simulink model "NeuromuscularModel_3R60CMG_3D"  (R2019b)
settings: Solver=ode15s  StartTime=0.0  StopTime=20  MaxStep=.001  MinStep=1e-34  RelTol=1e-5  AbsTol=1e-7  EnableMultiTasking=on
values from neighbouring files (symbols this model uses):
  animFrameRate = 30    [demorun.m]    (also in evaluateCost.m; optimize.m; optimizeCMG.m)
  dt_visual = 1/1000    (= 0.001)    [demorun.m]    (also in evaluateCost.m; optimize.m = 0.0333333333333; optimizeCMG.m)
  initialTargetAngle = 70*pi/180    (= 1.2217304764)    [setInit.m]
  LPreStimBFSHinit = initConditionsSagittal(12)    [assignInit.m]
  LPreStimGASinit = initConditionsSagittal(13)    [assignInit.m]
  LPreStimGLUinit = initConditionsSagittal(8)    [assignInit.m]
  LPreStimHABinit = initConditionsCoronal(6)    [assignInit.m]
  LPreStimHADinit = initConditionsCoronal(7)    [assignInit.m]
  LPreStimHAMinit = initConditionsSagittal(9)    [assignInit.m]
  LPreStimHFLinit = initConditionsSagittal(7)    [assignInit.m]
  LPreStimRFinit = initConditionsSagittal(10)    [assignInit.m]
  LPreStimSOLinit = initConditionsSagittal(14)    [assignInit.m]
  LPreStimTAinit = initConditionsSagittal(15)    [assignInit.m]
  LPreStimVASinit = initConditionsSagittal(11)    [assignInit.m]
  LTargetAngleInit = initConditionsSagittal(6)    [assignInit.m]
  LTargetAngleRInit = initConditionsCoronal(5)    [assignInit.m]
  RPreStimGLUinit = initConditionsSagittal(18)    [assignInit.m]
  RPreStimHABinit = initConditionsCoronal(9)    [assignInit.m]
  RPreStimHADinit = initConditionsCoronal(10)    [assignInit.m]
  RPreStimHAMinit = initConditionsSagittal(19)    [assignInit.m]
  RPreStimHFLinit = initConditionsSagittal(17)    [assignInit.m]
  RPreStimRFinit = initConditionsSagittal(20)    [assignInit.m]
  RTargetAngleInit = initConditionsSagittal(16)    [assignInit.m]
  RTargetAngleRInit = initConditionsCoronal(8)    [assignInit.m]
undefined symbols (not defined in the file or in its folder): DiscIntNeverNeededParam, g, hatLeftHipToCenterDistWidth, LongDelay, LongLoopDelay, MidDelay, ShortDelay, termination_height, thetaHATref, X, Y, Z
libraries: NeuroMuscularLibrary x96, nesl_utility x22, sm_lib x21, CMGlibrary x6, simulink x3
(part 2 of 3)

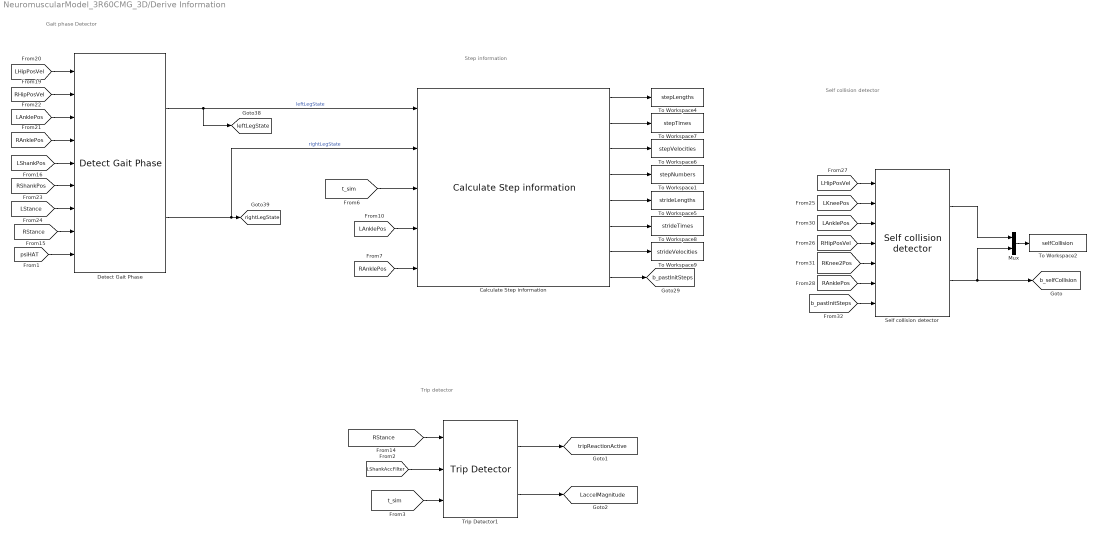
== system NeuromuscularModel_3R60CMG_3D/Derive Information ==
  note: Step information
  note: Self collision detector
  note: Gait phase Detector
  note: Trip detector
  Calculate Step information : NeuroMuscularLibrary/Calculate Step information  SystemSampleTime=-1  Latency=0  AutoFrameSizeCalculation=off
  Detect Gait Phase : NeuroMuscularLibrary/Detect Gait Phase  SystemSampleTime=-1  Latency=0  AutoFrameSizeCalculation=off
  Mux : Mux  Inputs=2
  Self collision detector : NeuroMuscularLibrary/Self collision detector  maxDist=0.02
  To Workspace1 : ToWorkspace  VariableName=stepNumbers  SaveFormat=Structure With Time  SampleTime=-1
  To Workspace2 : ToWorkspace  VariableName=selfCollision  SaveFormat=Structure With Time  SampleTime=dt_visual
  To Workspace4 : ToWorkspace  VariableName=stepLengths  SaveFormat=Structure With Time  SampleTime=-1
  To Workspace5 : ToWorkspace  VariableName=strideLengths  SaveFormat=Structure With Time  SampleTime=-1
  To Workspace6 : ToWorkspace  VariableName=stepVelocities  SaveFormat=Structure With Time  SampleTime=-1
  To Workspace7 : ToWorkspace  VariableName=stepTimes  SaveFormat=Structure With Time  SampleTime=-1
  To Workspace8 : ToWorkspace  VariableName=strideTimes  SaveFormat=Structure With Time  SampleTime=-1
  To Workspace9 : ToWorkspace  VariableName=strideVelocities  SaveFormat=Structure With Time  SampleTime=-1
  Trip Detector1 : CMGlibrary/Trip Detector  tripThreshold=tripDetectThreshold
  tag scope: LaccelMagnitude=global, b_pastInitSteps=global, b_selfCollision=global, leftLegState=global, rightLegState=global, tripReactionActive=global
  wires:
  [RAnklePos] -> Self collision detector/6
  [LAnklePos] -> Self collision detector/3
  Mux/1 -> To Workspace2/1
  [LStance] -> Detect Gait Phase/7
  [LKneePos] -> Self collision detector/2
  [LAnklePos] -> Detect Gait Phase/3
  Self collision detector/1 -> Mux/1
  [RStance] -> Detect Gait Phase/8
  [b_pastInitSteps] -> Self collision detector/7
  [RHipPosVel] -> Self collision detector/4
  Detect Gait Phase/2 -> Calculate Step information/2, [rightLegState]  "rightLegState"
  [LShankPos] -> Detect Gait Phase/5
  [RAnklePos] -> Detect Gait Phase/4
  [RHipPosVel] -> Detect Gait Phase/2
  Detect Gait Phase/1 -> Calculate Step information/1, [leftLegState]  "leftLegState"
  [RShankPos] -> Detect Gait Phase/6
  [LHipPosVel] -> Detect Gait Phase/1
  [psiHAT] -> Detect Gait Phase/9
  [RKnee2Pos] -> Self collision detector/5
  [LHipPosVel] -> Self collision detector/1
  Calculate Step information/1 -> To Workspace4/1
  [RAnklePos] -> Calculate Step information/5
  Calculate Step information/3 -> To Workspace6/1
  Calculate Step information/2 -> To Workspace7/1
  [t_sim] -> Calculate Step information/3
  Calculate Step information/8 -> [b_pastInitSteps]
  [LAnklePos] -> Calculate Step information/4
  Calculate Step information/4 -> To Workspace1/1
  Calculate Step information/5 -> To Workspace5/1
  Calculate Step information/6 -> To Workspace8/1
  Calculate Step information/7 -> To Workspace9/1
  [LShankAccFilter] -> Trip Detector1/2
  [t_sim] -> Trip Detector1/3
  [RStance] -> Trip Detector1/1
  Trip Detector1/1 -> [tripReactionActive]
  Trip Detector1/2 -> [LaccelMagnitude]
  Self collision detector/2 -> [b_selfCollision], Mux/2

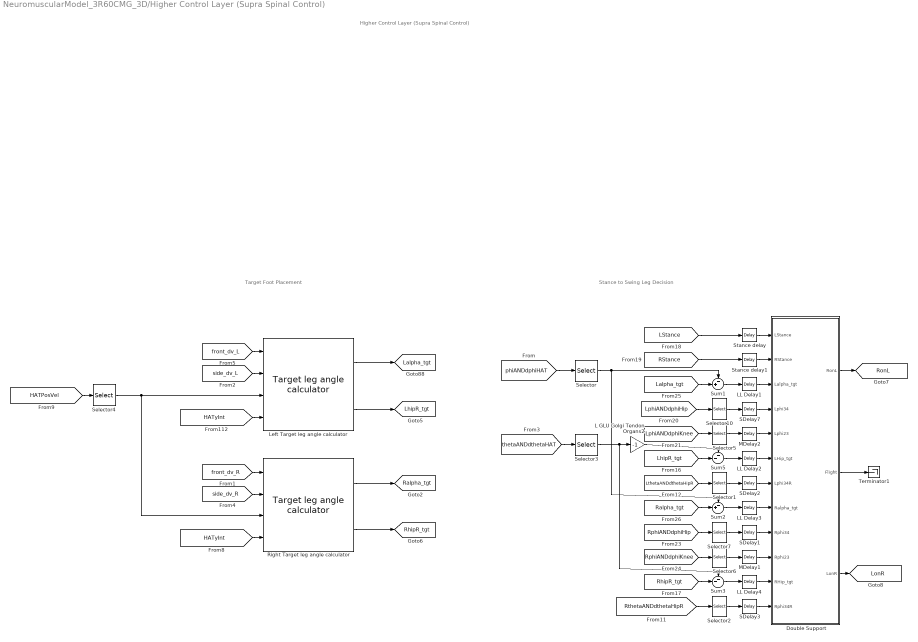
== system NeuromuscularModel_3R60CMG_3D/Higher Control Layer (Supra Spinal Control) ==
  note: Target Foot Placement
  note: Stance to Swing Leg Decision
  note: Higher Control Layer
      | (Supra Spinal Control)
  Double Support : Subsystem
  L GLU Golgi Tendon Organs2 : Gain  Gain=-1
  LL Delay1 : TransportDelay  DelayTime=LongLoopDelay/2  InitialOutput=initialTargetAngle
  LL Delay2 : TransportDelay  DelayTime=LongLoopDelay/2
  LL Delay3 : TransportDelay  DelayTime=LongLoopDelay/2  InitialOutput=initialTargetAngle
  LL Delay4 : TransportDelay  DelayTime=LongLoopDelay/2
  Left Target leg angle calculator : NeuroMuscularLibrary/Target leg angle calculator  simbiconLegAngle0=LsimbiconLegAngle0  simbiconGainD=LsimbiconGainD  simbiconGainV=LsimbiconGainV  simbiconLegAngle0_C=LsimbiconLegAngle0_C  simbiconGainD_C=LsimbiconGainD_C  simbiconGainV_C=LsimbiconGainV_C  headingGain=LheadingGain  headingIntGain=LheadingIntGain
  MDelay1 : TransportDelay  DelayTime=MidDelay
  MDelay2 : TransportDelay  DelayTime=MidDelay
  Right Target leg angle calculator : NeuroMuscularLibrary/Target leg angle calculator  simbiconLegAngle0=RsimbiconLegAngle0  simbiconGainD=RsimbiconGainD  simbiconGainV=RsimbiconGainV  simbiconLegAngle0_C=RsimbiconLegAngle0_C  simbiconGainD_C=RsimbiconGainD_C  simbiconGainV_C=RsimbiconGainV_C  headingGain=RheadingGain  headingIntGain=RheadingIntGain
  SDelay{1..3,7} (4 alike) : TransportDelay  DelayTime=ShortDelay
  Selector : Selector  InputPortWidth=2  IndexOptions=Index vector (dialog)  Indices=[1]  OutputSizes=1
  Selector{1..2,5..7,10} (6 alike) : Selector  InputPortWidth=2  IndexOptions=Index vector (dialog)  Indices=1  OutputSizes=1
  Selector3 : Selector  InputPortWidth=2  IndexOptions=Index vector (dialog)  Indices=[1]  OutputSizes=1
  Selector4 : Selector  InputPortWidth=6  IndexOptions=Index vector (dialog)  Indices=[2]  OutputSizes=1
  Stance delay : TransportDelay  DelayTime=MidDelay
  Stance delay1 : TransportDelay  DelayTime=MidDelay
  Sum1 : Sum  Inputs=-+|
  Sum2 : Sum  Inputs=-+|
  Sum3 : Sum  Inputs=--|
  Sum5 : Sum  Inputs=--|
  Terminator1 : Terminator
  tag scope: Lalpha_tgt=global, LhipR_tgt=global, LonR=global, Ralpha_tgt=global, RhipR_tgt=global, RonL=global
  wires:
  [LphiANDdphiHip] -> Selector10/1
  [LphiANDdphiKnee] -> Selector5/1
  Selector10/1 -> SDelay7/1
  Selector5/1 -> MDelay2/1
  [RphiANDdphiHip] -> Selector7/1
  [RphiANDdphiKnee] -> Selector6/1
  Selector7/1 -> SDelay1/1
  Selector6/1 -> MDelay1/1
  Stance delay/1 -> Double Support/1(LStance)
  Stance delay1/1 -> Double Support/2(RStance)
  [LStance] -> Stance delay/1
  [RStance] -> Stance delay1/1
  Double Support/2(Flight) -> Terminator1/1
  LL Delay1/1 -> Double Support/3(Lalpha_tgt)
  LL Delay3/1 -> Double Support/8(Ralpha_tgt)
  SDelay7/1 -> Double Support/4(Lphi34)
  SDelay1/1 -> Double Support/9(Rphi34)
  MDelay2/1 -> Double Support/5(Lphi23)
  MDelay1/1 -> Double Support/10(Rphi23)
  Sum1/1 -> LL Delay1/1
  [Lalpha_tgt] -> Sum1/2
  Selector/1 -> Sum2/1, Sum1/1
  [Ralpha_tgt] -> Sum2/2
  Sum2/1 -> LL Delay3/1
  [LthetaANDdthetaHipR] -> Selector1/1
  Selector1/1 -> SDelay2/1
  SDelay2/1 -> Double Support/7(Lphi34R)
  LL Delay2/1 -> Double Support/6(LHip_tgt)
  Sum5/1 -> LL Delay2/1
  [LhipR_tgt] -> Sum5/2
  Selector3/1 -> L GLU Golgi Tendon Organs2/1, Sum3/1
  L GLU Golgi Tendon Organs2/1 -> Sum5/1
  [RthetaANDdthetaHipR] -> Selector2/1
  Selector2/1 -> SDelay3/1
  SDelay3/1 -> Double Support/12(Rphi34R)
  LL Delay4/1 -> Double Support/11(RHip_tgt)
  Sum3/1 -> LL Delay4/1
  [RhipR_tgt] -> Sum3/2
  [phiANDdphiHAT] -> Selector/1
  [thetaANDdthetaHAT] -> Selector3/1
  Right Target leg angle calculator/2 -> [RhipR_tgt]
  Right Target leg angle calculator/1 -> [Ralpha_tgt]
  Left Target leg angle calculator/2 -> [LhipR_tgt]
  Left Target leg angle calculator/1 -> [Lalpha_tgt]
  [side_dv_R] -> Right Target leg angle calculator/2
  [side_dv_L] -> Left Target leg angle calculator/2
  [front_dv_R] -> Right Target leg angle calculator/1
  [front_dv_L] -> Left Target leg angle calculator/1
  Double Support/1(RonL) -> [RonL]
  Double Support/3(LonR) -> [LonR]
  [HATyInt] -> Left Target leg angle calculator/4
  [HATyInt] -> Right Target leg angle calculator/4
  [HATPosVel] -> Selector4/1
  Selector4/1 -> Right Target leg angle calculator/3, Left Target leg angle calculator/3

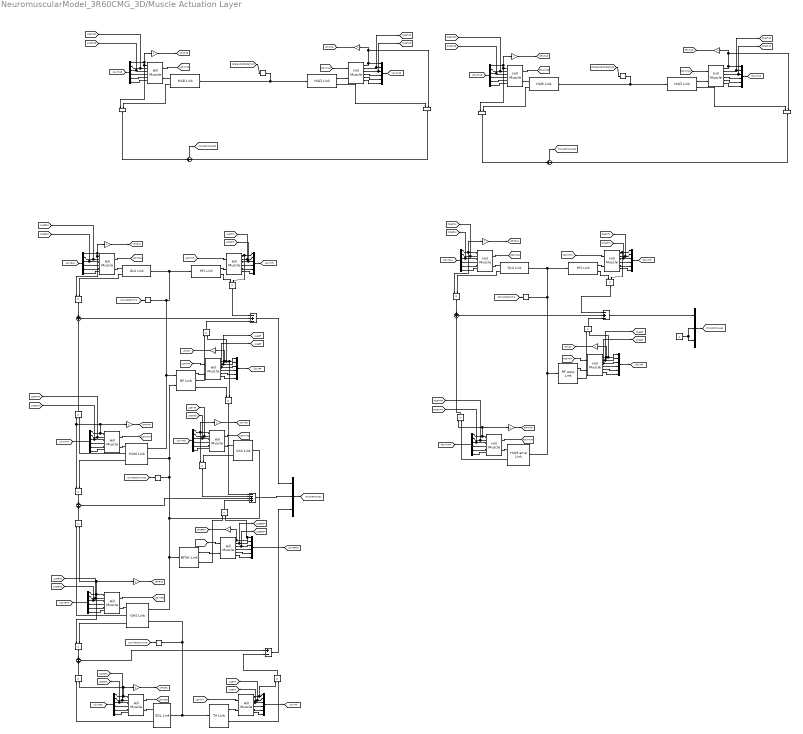
== system NeuromuscularModel_3R60CMG_3D/Muscle Actuation Layer ==
  note: Right Hip Joint
  note: Right Knee Joint
  note: Left Hip Joint
  note: Left Knee Joint
  note: Left Ankle Joint
  note: Left Leg
  note: Right Leg
  note: Body Mechanics Layer
      | Interface (Left Hip Joint)
  note: Muscle Actuation Layer
      | (Coronal Plane)
  note: Muscle Actuation Layer
      | (Sagittal Plane)
  note: Body Mechanics Layer
      | Interface (Right Hip Joint)
  Add1 : Sum  Inputs=-+-
  Add2 : Sum  Inputs=-+-
  Add5 : Sum  Inputs=--++
  Add6 : Sum  Inputs=+-
  Constant : Constant  Value=0
  L  TA Link : NeuroMuscularLibrary/TA Link  SystemSampleTime=-1  Latency=0  AutoFrameSizeCalculation=off
  L BFSH Golgi Tendon Organs : Gain
  L BFSH Link : NeuroMuscularLibrary/BFSH Link  SystemSampleTime=-1  Latency=0  AutoFrameSizeCalculation=off
  L BFSH Muscle : NeuroMuscularLibrary/Hill Muscle  Fmax=FmaxBFSH  lopt=loptBFSH  vmax=vmaxBFSH  lslack=lslackBFSH
  L GAS Golgi Tendon Organs : Gain
  L GAS Link : NeuroMuscularLibrary/GAS Link  SystemSampleTime=-1  Latency=0  AutoFrameSizeCalculation=off
  L GAS Muscle : NeuroMuscularLibrary/Hill Muscle  Fmax=FmaxGAS  lopt=loptGAS  vmax=vmaxGAS  lslack=lslackGAS
  L GLU Golgi Tendon Organs : Gain
  L GLU Link : NeuroMuscularLibrary/GLU Link  SystemSampleTime=-1  Latency=0  AutoFrameSizeCalculation=off
  L GLU Muscle : NeuroMuscularLibrary/Hill Muscle  Fmax=FmaxGLU  lopt=loptGLU  vmax=vmaxGLU  lslack=lslackGLU
  L HAB Golgi Tendon Organs : Gain
  L HAB Link : NeuroMuscularLibrary/HAB Link  SystemSampleTime=-1  Latency=0  AutoFrameSizeCalculation=off
  L HAB Muscle : NeuroMuscularLibrary/Hill Muscle  Fmax=FmaxHAB  lopt=loptHAB  vmax=vmaxHAB  lslack=lslackHAB
  L HAD Golgi Tendon Organs : Gain
  L HAD Link : NeuroMuscularLibrary/HAD Link  SystemSampleTime=-1  Latency=0  AutoFrameSizeCalculation=off
  L HAD Muscle : NeuroMuscularLibrary/Hill Muscle  Fmax=FmaxHAD  lopt=loptHAD  vmax=vmaxHAD  lslack=lslackHAD
  L HAM Golgi Tendon Organs : Gain
  L HAM Link : NeuroMuscularLibrary/HAM Link  SystemSampleTime=-1  Latency=0  AutoFrameSizeCalculation=off
  L HAM Muscle : NeuroMuscularLibrary/Hill Muscle  Fmax=FmaxHAM  lopt=loptHAM  vmax=vmaxHAM  lslack=lslackHAM
  L HFL Link : NeuroMuscularLibrary/HFL Link  SystemSampleTime=-1  Latency=0  AutoFrameSizeCalculation=off
  L HFL Muscle : NeuroMuscularLibrary/Hill Muscle  Fmax=FmaxHFL  lopt=loptHFL  vmax=vmaxHFL  lslack=lslackHFL
  L RF Golgi Tendon Organs : Gain
  L RF Link : NeuroMuscularLibrary/RF Link  SystemSampleTime=-1  Latency=0  AutoFrameSizeCalculation=off
  L RF Muscle : NeuroMuscularLibrary/Hill Muscle  Fmax=FmaxRF  lopt=loptRF  vmax=vmaxRF  lslack=lslackRF
  L SOL Golgi Tendon Organs : Gain
  L SOL Link : NeuroMuscularLibrary/SOL Link  SystemSampleTime=-1  Latency=0  AutoFrameSizeCalculation=off
  L SOL Muscle : NeuroMuscularLibrary/Hill Muscle  Fmax=FmaxSOL  lopt=loptSOL  vmax=vmaxSOL  lslack=lslackSOL
  L TA Muscle : NeuroMuscularLibrary/Hill Muscle  Fmax=FmaxTA  lopt=loptTA  vmax=vmaxTA  lslack=lslackTA
  L VAS Golgi Tendon Organs : Gain
  L VAS Link : NeuroMuscularLibrary/VAS Link  SystemSampleTime=-1  Latency=0  AutoFrameSizeCalculation=off
  L VAS Muscle : NeuroMuscularLibrary/Hill Muscle  Fmax=FmaxVAS  lopt=loptVAS  vmax=vmaxVAS  lslack=lslackVAS
  Mux : Mux  Inputs=3
  Mux1 : Mux  Inputs=3
  Mux{2..10,15..17,19..23} (17 alike) : Mux  Inputs=6
  Product{1..2,26..27} (4 alike) : Product  RndMeth=Zero
  R GLU Golgi Tendon Organs : Gain
  R GLU Link : NeuroMuscularLibrary/GLU Link  SystemSampleTime=-1  Latency=0  AutoFrameSizeCalculation=off
  R GLU amp Muscle : NeuroMuscularLibrary/Hill Muscle  Fmax=FmaxGLUamp  lopt=loptGLUamp  vmax=vmaxGLUamp  lslack=lslackGLUamp
  R HAB Golgi Tendon Organs : Gain
  R HAB Link : NeuroMuscularLibrary/HAB Link  SystemSampleTime=-1  Latency=0  AutoFrameSizeCalculation=off
  R HAB amp Muscle : NeuroMuscularLibrary/Hill Muscle  Fmax=FmaxHABamp  lopt=loptHABamp  vmax=vmaxHABamp  lslack=lslackHABamp
  R HAD Golgi Tendon Organs : Gain
  R HAD Link : NeuroMuscularLibrary/HAD Link  SystemSampleTime=-1  Latency=0  AutoFrameSizeCalculation=off
  R HAD Muscle : NeuroMuscularLibrary/Hill Muscle  Fmax=FmaxHADamp  lopt=loptHADamp  vmax=vmaxHADamp  lslack=lslackHADamp
  R HAM Golgi Tendon Organs : Gain
  R HAM amp Link : NeuroMuscularLibrary/HAM amp Link  SystemSampleTime=-1  Latency=0  AutoFrameSizeCalculation=off
  R HAM amp Muscle : NeuroMuscularLibrary/Hill Muscle  Fmax=FmaxHAMamp  lopt=loptHAMamp  vmax=vmaxHAMamp  lslack=lslackHAMamp
  R HFL  Link : NeuroMuscularLibrary/HFL Link  SystemSampleTime=-1  Latency=0  AutoFrameSizeCalculation=off
  R HFL amp Muscle : NeuroMuscularLibrary/Hill Muscle  Fmax=FmaxHFLamp  lopt=loptHFLamp  vmax=vmaxHFLamp  lslack=lslackHFLamp
  R RF Golgi Tendon Organs : Gain
  R RF amp Link : NeuroMuscularLibrary/RF amp Link  SystemSampleTime=-1  Latency=0  AutoFrameSizeCalculation=off
  R RF amp Muscle : NeuroMuscularLibrary/Hill Muscle  Fmax=FmaxRFamp  lopt=loptRFamp  vmax=vmaxRFamp  lslack=lslackRFamp
  Selector{1,4..8} (6 alike) : Selector  InputPortWidth=2  IndexOptions=Index vector (dialog)  Indices=1  OutputSizes=1
  Sum{1,3..4,8} (4 alike) : Sum  Inputs=+|+
  Sum2 : Sum  Inputs=+-
  Sum25 : Sum  Inputs=+-
  tau = r*F{1..11,18..21,24} (16 alike) : Product
  tag scope: LFmBFSH=global, LFmGAS=global, LFmGLU=global, LFmHAB=global, LFmHAD=global, LFmHAM=global, LFmRF=global, LFmSOL=global, LFmVAS=global, LLceBFSH=global, LLceGAS=global, LLceGLU=global, LLceHAB=global, LLceHAD=global, LLceHAM=global, LLceHFL=global, LLceRF=global, LLceSOL=global, LLceTA=global, LLceVAS=global, LMuscleTorques=global, LMuscleTorquesR=global, LVceBFSH=global, LVceGAS=global, LVceGLU=global, LVceHAB=global, LVceHAD=global, LVceHAM=global, LVceHFL=global, LVceRF=global, LVceSOL=global, LVceTA=global, LVceVAS=global, LdynBFSH=global, LdynGAS=global, LdynGLU=global, LdynHAB=global, LdynHAD=global, LdynHAM=global, LdynHFL=global, LdynRF=global, LdynSOL=global, LdynTA=global, LdynVAS=global, RFmGLU=global, RFmHAB=global, RFmHAD=global, RFmHAM=global, RFmRF=global, RLceGLU=global, RLceHAB=global, RLceHAD=global, RLceHAM=global, RLceHFL=global, RLceRF=global, RMuscleTorques=global, RMuscleTorquesR=global, RVceGLU=global, RVceHAB=global, RVceHAD=global, RVceHAM=global, RVceHFL=global, RVceRF=global, RdynGLU=global, RdynHAB=global, RdynHAD=global, RdynHAM=global, RdynHFL=global, RdynRF=global
  wires:
  R HAM amp Link/1 -> R HAM amp Muscle/2
  R HAM amp Link/2 -> tau = r*F9/2
  R HAM amp Muscle/5 -> Mux7/5
  Mux7/1 -> [RdynHAM]
  R HAM amp Muscle/3 -> [RVceHAM], Mux7/3
  R HAM amp Muscle/4 -> Mux7/4
  [RphiANDdphiHip] -> Selector1/1
  Selector1/1 -> R HAM amp Link/1, R RF amp Link/1, R GLU Link/1, R HFL  Link/1
  Add2/1 -> Mux/1
  R GLU Link/1 -> R GLU amp Muscle/2
  [RStimGLU] -> R GLU amp Muscle/1
  R GLU amp Muscle/5 -> Mux9/5
  R GLU amp Muscle/2 -> [RLceGLU], Mux9/2
  R GLU amp Muscle/3 -> [RVceGLU], Mux9/3
  R GLU amp Muscle/4 -> Mux9/4
  R GLU Link/2 -> tau = r*F10/2
  R GLU amp Muscle/1 -> Mux9/1, R GLU Golgi Tendon Organs/1, tau = r*F10/1
  R GLU Golgi Tendon Organs/1 -> [RFmGLU]
  R HFL  Link/1 -> R HFL amp Muscle/2
  [RStimHFL] -> R HFL amp Muscle/1
  R HFL amp Muscle/5 -> Mux10/5
  Mux10/1 -> [RdynHFL]
  R HFL amp Muscle/4 -> Mux10/4
  R HFL amp Muscle/3 -> [RVceHFL], Mux10/3
  R HFL  Link/2 -> tau = r*F11/1
  R HFL amp Muscle/1 -> Mux10/1, tau = r*F11/2
  R HAM Golgi Tendon Organs/1 -> [RFmHAM]
  [RStimHAM] -> R HAM amp Muscle/1
  tau = r*F9/1 -> Sum8/2  "HAM"
  tau = r*F10/1 -> Sum8/1  "GLU"
  tau = r*F11/1 -> Add2/1  "HFL"
  R HAM amp Muscle/1 -> tau = r*F9/1, R HAM Golgi Tendon Organs/1, Mux7/1
  Sum8/1 -> Add2/2  "Hip Extension Moment"
  Mux9/1 -> [RdynGLU]
  Mux/1 -> [RMuscleTorques]
  L HAM Link/1 -> L HAM Muscle/2
  L HAM Link/2 -> tau = r*F18/2
  L HAM Muscle/5 -> Mux8/5
  Mux8/1 -> [LdynHAM]
  L HAM Muscle/3 -> [LVceHAM], Mux8/3
  L HAM Muscle/4 -> Mux8/4
  [LphiANDdphiHip] -> Selector4/1
  Selector4/1 -> L GLU Link/1, L HFL Link/1, L RF Link/1, L HAM Link/1
  Add1/1 -> Mux1/1
  L GLU Link/1 -> L GLU Muscle/2
  [LStimGLU] -> L GLU Muscle/1
  L GLU Muscle/5 -> Mux15/5
  L GLU Muscle/2 -> Mux15/2, [LLceGLU]
  L GLU Muscle/3 -> Mux15/3, [LVceGLU]
  L GLU Muscle/4 -> Mux15/4
  L GLU Link/2 -> tau = r*F1/2
  L GLU Muscle/1 -> Mux15/1, L GLU Golgi Tendon Organs/1, tau = r*F1/1
  L GLU Golgi Tendon Organs/1 -> [LFmGLU]
  L HFL Link/1 -> L HFL Muscle/2
  [LStimHFL] -> L HFL Muscle/1
  L HFL Muscle/5 -> Mux2/5
  Mux2/1 -> [LdynHFL]
  L HFL Muscle/4 -> Mux2/4
  L HFL Muscle/3 -> [LVceHFL], Mux2/3
  L HFL Link/2 -> tau = r*F2/1
  L HFL Muscle/1 -> Mux2/1, tau = r*F2/2
  L HAM Golgi Tendon Organs/1 -> [LFmHAM]
  [LStimHAM] -> L HAM Muscle/1
  L VAS Link/1 -> L VAS Muscle/2
  L VAS Muscle/5 -> Mux3/5
  Mux3/1 -> [LdynVAS]
  L VAS Muscle/2 -> [LLceVAS], Mux3/2
  L VAS Muscle/3 -> [LVceVAS], Mux3/3
  L VAS Muscle/4 -> Mux3/4
  L VAS Muscle/1 -> L VAS Golgi Tendon Organs/1, Mux3/1, tau = r*F4/1
  L VAS Golgi Tendon Organs/1 -> [LFmVAS]
  L VAS Link/2 -> tau = r*F4/2
  L HAM Link/3 -> tau = r*F5/2
  Sum1/1 -> Add5/3  "Knee Flexion Torque"
  [LStimVAS] -> L VAS Muscle/1
  [LphiANDdphiKnee] -> Selector6/1
  L SOL Muscle/1 -> L SOL Golgi Tendon Organs/1, tau = r*F3/2, Mux5/1
  L SOL Muscle/5 -> Mux5/5
  Mux5/1 -> [LdynSOL]
  L SOL Muscle/3 -> [LVceSOL], Mux5/3
  L SOL Muscle/4 -> Mux5/4
  L SOL Link/2 -> tau = r*F3/1
  L SOL Link/1 -> L SOL Muscle/2
  L SOL Golgi Tendon Organs/1 -> [LFmSOL]
  [LStimSOL] -> L SOL Muscle/1
  Selector5/1 -> L GAS Link/2, L  TA Link/1, L SOL Link/1
  [LphiANDdphiAnkle] -> Selector5/1
  Add6/1 -> Mux1/3
  L  TA Link/1 -> L TA Muscle/2
  L TA Muscle/1 -> tau = r*F6/1, Mux6/1
  L TA Muscle/5 -> Mux6/5
  Mux6/1 -> [LdynTA]
  L TA Muscle/4 -> Mux6/4
  L TA Muscle/3 -> Mux6/3, [LVceTA]
  [LStimTA] -> L TA Muscle/1
  L  TA Link/2 -> tau = r*F6/2
  tau = r*F6/1 -> Add6/2
  L GAS Link/1 -> L GAS Muscle/2
  Selector6/1 -> L GAS Link/1, L BFSH Link/1, L VAS Link/1, L RF Link/2, L HAM Link/2
  L GAS Muscle/5 -> Mux4/5
  Mux4/1 -> [LdynGAS]
  L GAS Muscle/2 -> [LLceGAS], Mux4/2
  L GAS Muscle/3 -> [LVceGAS], Mux4/3
  L GAS Muscle/4 -> Mux4/4
  L GAS Link/2 -> tau = r*F7/1
  [LStimGAS] -> L GAS Muscle/1
  tau = r*F3/1 -> Sum3/2
  Sum3/1 -> Add6/1
  L GAS Link/3 -> tau = r*F8/2
  tau = r*F8/1 -> Sum3/1
  L GAS Muscle/1 -> Mux4/1, tau = r*F7/2, L GAS Golgi Tendon Organs/1, tau = r*F8/1
  L GAS Golgi Tendon Organs/1 -> [LFmGAS]
  tau = r*F18/1 -> Sum4/2  "HAM"
  tau = r*F1/1 -> Sum4/1  "GLU"
  tau = r*F2/1 -> Add1/1  "HFL"
  L HAM Muscle/1 -> tau = r*F5/1, tau = r*F18/1, L HAM Golgi Tendon Organs/1, Mux8/1
  Sum4/1 -> Add1/2  "Hip Extension Moment"
  tau = r*F7/1 -> Sum1/2  "GAS"
  tau = r*F5/1 -> Sum1/1  "HAM"
  tau = r*F4/1 -> Add5/2  "VAS"
  L TA Muscle/2 -> [LLceTA], Mux6/2
  Mux15/1 -> [LdynGLU]
  Mux1/1 -> [LMuscleTorques]
  L GLU Muscle/6 -> Mux15/6
  L HFL Muscle/6 -> Mux2/6
  L HAM Muscle/6 -> Mux8/6
  L VAS Muscle/6 -> Mux3/6
  L GAS Muscle/6 -> Mux4/6
  L SOL Muscle/6 -> Mux5/6
  L TA Muscle/6 -> Mux6/6
  R HAM amp Muscle/6 -> Mux7/6
  R HFL amp Muscle/6 -> Mux10/6
  R GLU amp Muscle/6 -> Mux9/6
  R HFL amp Muscle/2 -> [RLceHFL], Mux10/2
  R HAM amp Muscle/2 -> [RLceHAM], Mux7/2
  L HFL Muscle/2 -> [LLceHFL], Mux2/2
  L HAM Muscle/2 -> [LLceHAM], Mux8/2
  L SOL Muscle/2 -> [LLceSOL], Mux5/2
  L BFSH Muscle/3 -> [LVceBFSH], Mux16/3
  [LStimBFSH] -> L BFSH Muscle/1
  L BFSH Link/2 -> tau = r*F19/1
  L BFSH Golgi Tendon Organs/1 -> [LFmBFSH]
  L BFSH Muscle/6 -> Mux16/6
  L BFSH Muscle/4 -> Mux16/4
  L BFSH Link/1 -> L BFSH Muscle/2
  Mux16/1 -> [LdynBFSH]
  L BFSH Muscle/2 -> [LLceBFSH], Mux16/2
  L BFSH Muscle/5 -> Mux16/5
  L BFSH Muscle/1 -> tau = r*F19/2, Mux16/1, L BFSH Golgi Tendon Organs/1
  tau = r*F19/1 -> Add5/4  "BFSH"
  L RF Muscle/3 -> [LVceRF], Mux17/3
  [LStimRF] -> L RF Muscle/1
  L RF Link/3 -> tau = r*F20/2
  L RF Golgi Tendon Organs/1 -> [LFmRF]
  L RF Muscle/6 -> Mux17/6
  L RF Muscle/4 -> Mux17/4
  L RF Link/1 -> L RF Muscle/2
  Mux17/1 -> [LdynRF]
  L RF Muscle/2 -> [LLceRF], Mux17/2
  L RF Muscle/5 -> Mux17/5
  L RF Muscle/1 -> tau = r*F21/2, Mux17/1, tau = r*F20/1, L RF Golgi Tendon Organs/1
  L RF Link/2 -> tau = r*F21/1
  tau = r*F21/1 -> Add1/3  "RF"
  tau = r*F20/1 -> Add5/1  "RF"
  [RStimRF] -> R RF amp Muscle/1
  R RF amp Muscle/3 -> [RVceRF], Mux19/3
  R RF amp Muscle/4 -> Mux19/4
  R RF amp Muscle/6 -> Mux19/6
  R RF amp Muscle/5 -> Mux19/5
  R RF amp Muscle/2 -> [RLceRF], Mux19/2
  R RF amp Muscle/1 -> tau = r*F24/2, Mux19/1, R RF Golgi Tendon Organs/1
  Mux19/1 -> [RdynRF]
  R RF amp Link/2 -> tau = r*F24/1
  R RF Golgi Tendon Organs/1 -> [RFmRF]
  R RF amp Link/1 -> R RF amp Muscle/2
  tau = r*F24/1 -> Add2/3  "RF"
  Product27/1 -> Sum25/2
  L HAD Link/2 -> Product27/1
  Selector7/1 -> L HAB Link/1, L HAD Link/1
  Product26/1 -> Sum25/1
  L HAB Muscle/6 -> Mux20/6
  L HAB Muscle/1 -> Product26/1, Mux20/1, L HAB Golgi Tendon Organs/1
  L HAB Golgi Tendon Organs/1 -> [LFmHAB]
  L HAB Muscle/4 -> Mux20/4
  L HAB Muscle/2 -> Mux20/2, [LLceHAB]
  L HAB Muscle/5 -> Mux20/5
  L HAB Link/1 -> L HAB Muscle/2
  L HAB Link/2 -> Product26/2
  L HAB Muscle/3 -> Mux20/3, [LVceHAB]
  [LStimHAB] -> L HAB Muscle/1
  Mux20/1 -> [LdynHAB]
  [LthetaANDdthetaHipR] -> Selector7/1
  L HAD Link/1 -> L HAD Muscle/2
  [LStimHAD] -> L HAD Muscle/1
  L HAD Golgi Tendon Organs/1 -> [LFmHAD]
  L HAD Muscle/2 -> Mux21/2, [LLceHAD]
  L HAD Muscle/1 -> Mux21/1, Product27/2, L HAD Golgi Tendon Organs/1
  L HAD Muscle/3 -> [LVceHAD], Mux21/3
  L HAD Muscle/4 -> Mux21/4
  L HAD Muscle/5 -> Mux21/5
  L HAD Muscle/6 -> Mux21/6
  Mux21/1 -> [LdynHAD]
  Sum25/1 -> [LMuscleTorquesR]
  R HAD Muscle/6 -> Mux23/6
  Selector8/1 -> R HAB Link/1, R HAD Link/1
  R HAD Link/2 -> Product2/1
  R HAD Golgi Tendon Organs/1 -> [RFmHAD]
  [RStimHAD] -> R HAD Muscle/1
  Mux23/1 -> [RdynHAD]
  Sum2/1 -> [RMuscleTorquesR]
  Mux22/1 -> [RdynHAB]
  R HAB Golgi Tendon Organs/1 -> [RFmHAB]
  Product1/1 -> Sum2/1
  Product2/1 -> Sum2/2
  R HAD Muscle/5 -> Mux23/5
  R HAD Muscle/2 -> Mux23/2, [RLceHAD]
  R HAD Muscle/3 -> [RVceHAD], Mux23/3
  R HAD Link/1 -> R HAD Muscle/2
  [RthetaANDdthetaHipR] -> Selector8/1
  R HAD Muscle/1 -> Mux23/1, Product2/2, R HAD Golgi Tendon Organs/1
  R HAB Link/2 -> Product1/2
  R HAB amp Muscle/5 -> Mux22/5
  R HAB amp Muscle/2 -> Mux22/2, [RLceHAB]
  R HAD Muscle/4 -> Mux23/4
  R HAB Link/1 -> R HAB amp Muscle/2
  R HAB amp Muscle/4 -> Mux22/4
  R HAB amp Muscle/3 -> Mux22/3, [RVceHAB]
  R HAB amp Muscle/6 -> Mux22/6
  R HAB amp Muscle/1 -> Product1/1, Mux22/1, R HAB Golgi Tendon Organs/1
  [RStimHAB] -> R HAB amp Muscle/1
  Add5/1 -> Mux1/2
  Constant/1 -> Mux/3, Mux/2

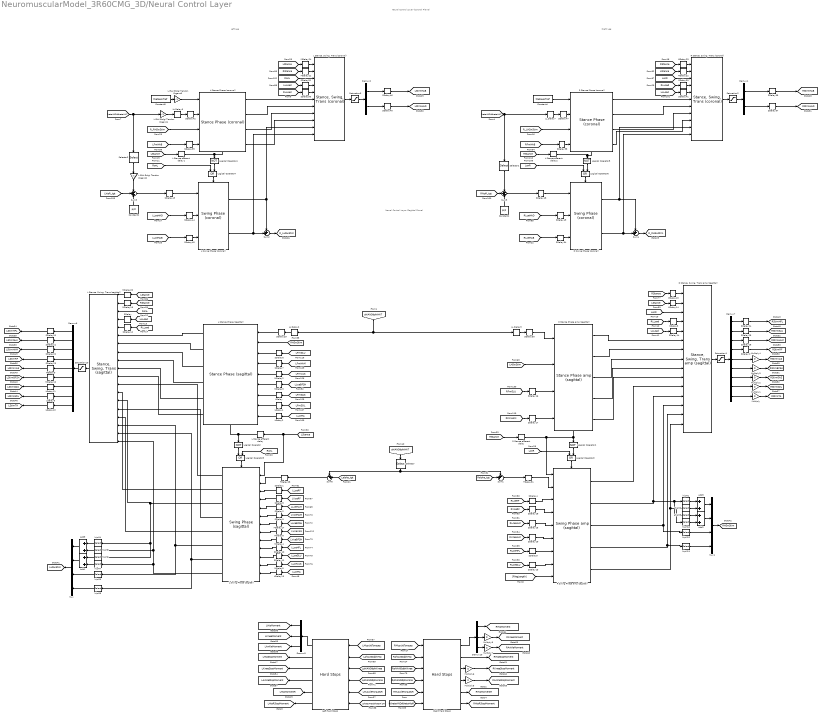
== system NeuromuscularModel_3R60CMG_3D/Neural Control Layer ==
  note: Neural Control Layer
      | (Sagittal Plane)
  note: Neural Control Layer
      | (Coronal Plane)
  note: Right Leg
  note: Left Leg
  Add{1..3,9} (4 alike) : Sum  Inputs=2
  Constant1 : Constant  Value=pi/2
  Constant2 : Constant  Value=pi/2
  Constant3 : Constant  Value=thetaHATref
  Constant4 : Constant  Value=thetaHATref
  Demux1 : Demux  Outputs=2
  Demux10 : Demux  Outputs=3
  Demux2 : Demux  Outputs=2
  Demux6 : Demux  Outputs=9
  Demux7 : Demux  Outputs=9
  Demux8 : Demux  Outputs=3
  L GLU Golgi Tendon Organs1 : Gain  Gain=-1
  L GLU Golgi Tendon Organs2 : Gain  Gain=-1
  L GLU Golgi Tendon Organs3 : Gain  Gain=-1
  L Stance afferent delay : TransportDelay  DelayTime=MidDelay
  L Stance afferent delay1 : TransportDelay  DelayTime=MidDelay
  L Stance afferent delay2 : TransportDelay  DelayTime=MidDelay
  L Stance Phase (coronal) : NeuroMuscularLibrary/Stance Phase (coronal)  PreStimHABst=LPreStimHABst  PreStimHADst=LPreStimHADst  GainFHABst=LGainFHABst  GainPhiHATHABst=LGainPhiHATHABst  GainDphiHATHABst=LGainDphiHATHABst  GainPhiHATHADst=LGainPhiHATHADst  GainDphiHATHADst=LGainDphiHATHADst  GainSHABcHABst=LGainSHABcHABst  GainSHADcHADst=LGainSHADcHADst
  L Stance Phase (sagittal) : NeuroMuscularLibrary/Stance Phase (sagittal)  PreStimHFLst=LPreStimHFLst  PreStimGLUst=LPreStimGLUst  PreStimHAMst=LPreStimHAMst  PreStimRFst=LPreStimRFst  PreStimVASst=LPreStimVASst  PreStimBFSHst=LPreStimBFSHst  PreStimGASst=LPreStimGASst  PreStimSOLst=LPreStimSOLst  PreStimTAst=LPreStimTAst  GainFGLUst=LGainFGLUst  GainFVASst=LGainFVASst  GainFSOLst=LGainFSOLst  GainFHAMst=LGainFHAMst  LceOffsetBFSHVASst=LLceOffsetBFSHVASst  GainLBFSHVASst=LGainLBFSHVASst  LceOffsetBFSHst=LLceOffsetBFSHst  GainLBFSHst=LGainLBFSHst  GainFGASst=LGainFGASst  phiHATref=phiHATref  GainPhiHATHFLst=LGainPhiHATHFLst  GainDphiHATHFLst=LGainDphiHATHFLst  GainPhiHATGLUst=LGainPhiHATGLUst  GainDphiHATGLUst=LGainDphiHATGLUst  GainSGLUHAMst=LGainSGLUHAMst  GainSGLUcHFLst=LGainSGLUcHFLst  GainSHAMcHFLst=LGainSHAMcHFLst  GainSHFLcGLUst=LGainSHFLcGLUst  GainSRFcGLUst=LGainSRFcGLUst  LceOffsetTAst=LLceOffsetTAst  GainLTAst=LGainLTAst  GainFSOLTAst=LGainFSOLTAst
  "L Stance, Swing, Trans (coronal)" : NeuroMuscularLibrary/Stance, Swing, Trans (coronal)  transSupst_C=LtransSupst_C  transsw_C=Ltranssw_C
  "L Stance, Swing, Trans (sagittal)" : NeuroMuscularLibrary/Stance, Swing, Trans (sagittal)  transSupst=LtransSupst  transsw=Ltranssw
  L Swing Phase (coronal) : NeuroMuscularLibrary/Swing Phase (coronal)  PreStimHABsw=LPreStimHABsw  PreStimHADsw=LPreStimHADsw  GainLHABsw=LGainLHABsw  GainLHADsw=LGainLHADsw
  L Swing Phase (sagittal) : NeuroMuscularLibrary/Swing Phase (sagittal)  PreStimHFLsw=LPreStimHFLsw  PreStimGLUsw=LPreStimGLUsw  PreStimHAMsw=LPreStimHAMsw  PreStimRFsw=LPreStimRFsw  PreStimVASsw=LPreStimVASsw  PreStimBFSHsw=LPreStimBFSHsw  PreStimGASsw=LPreStimGASsw  PreStimSOLsw=LPreStimSOLsw  PreStimTAsw=LPreStimTAsw  GainLTAsw=LGainLTAsw  LceOffsetTAsw=LLceOffsetTAsw  GainLRFHFLsw=LGainLRFHFLsw  GainVRFHFLsw=LGainVRFHFLsw  GainLHAMGLUsw=LGainLHAMGLUsw  GainVHAMGLUsw=LGainVHAMGLUsw  GainVRFBFSHsw=LGainVRFBFSHsw  GainVVASRFsw=LGainVVASRFsw  GainVBFSHsw=LGainVBFSHsw  GainLHAMsw=LGainLHAMsw  GainSHAMBFSHsw=LGainSHAMBFSHsw  GainSHAMGASsw=LGainSHAMGASsw  SHAMthresholdsw=LSHAMthresholdsw  GainLHFLsw=LGainLHFLsw  GainLGLUsw=LGainLGLUsw  LceOffsetVASsw=LLceOffsetVASsw  GainLVASsw=LGainLVASsw  legLengthClr=LlegLengthClr  deltaLegAngleThr=LdeltaLegAngleThr
  LDelay : TransportDelay  DelayTime=LongDelay
  LDelay1 : TransportDelay  DelayTime=LongDelay
  LDelay10 : TransportDelay  DelayTime=LongDelay  InitialOutput=LPreStimTAinit
  LDelay11 : TransportDelay  DelayTime=LongDelay  InitialOutput=LPreStimGASinit
  LDelay13 : TransportDelay  DelayTime=LongDelay  InitialOutput=1
  LDelay2 : TransportDelay  DelayTime=LongDelay  InitialOutput=1
  LDelay9 : TransportDelay  DelayTime=LongDelay  InitialOutput=LPreStimSOLinit
  LL Delay{2..3,6..7} (4 alike) : TransportDelay  DelayTime=LongLoopDelay/2
  Left Hard Stops : NeuroMuscularLibrary/Hard Stops  SystemSampleTime=-1  Latency=0  AutoFrameSizeCalculation=off
  Logical Operator{,1,4..5} (4 alike) : Logic  Operator=NOT  AllPortsSameDT=off  OutDataTypeStr=boolean
  Logical Operator{2..3,6..7} (4 alike) : Logic  Operator=OR  AllPortsSameDT=off  OutDataTypeStr=boolean
  MDelay10 : TransportDelay  DelayTime=MidDelay  InitialOutput=LPreStimBFSHinit
  MDelay{2,4,8,13..14,19..24} (11 alike) : TransportDelay  DelayTime=MidDelay
  MDelay17 : TransportDelay  DelayTime=MidDelay  InitialOutput=1
  MDelay3 : TransportDelay  DelayTime=MidDelay  InitialOutput=1
  MDelay5 : TransportDelay  DelayTime=MidDelay  InitialOutput=1
  MDelay9 : TransportDelay  DelayTime=MidDelay  InitialOutput=LPreStimVASinit
  Multiply{,1..8} (9 alike) : Gain  Gain=0
  Mux : Mux
  Mux1 : Mux
  R Stance afferent delay : TransportDelay  DelayTime=MidDelay
  R Stance Phase (coronal) : NeuroMuscularLibrary/Stance Phase (coronal)  PreStimHABst=RPreStimHABst  PreStimHADst=RPreStimHADst  GainFHABst=RGainFHABst  GainPhiHATHABst=RGainPhiHATHABst  GainDphiHATHABst=RGainDphiHATHABst  GainPhiHATHADst=RGainPhiHATHADst  GainDphiHATHADst=RGainDphiHATHADst  GainSHABcHABst=RGainSHABcHABst  GainSHADcHADst=RGainSHADcHADst
  R Stance Phase amp (sagittal) : NeuroMuscularLibrary/Stance Phase amp (sagittal)  PreStimHFLst=RPreStimHFLst  PreStimGLUst=RPreStimGLUst  PreStimHAMst=RPreStimHAMst  PreStimRFst=RPreStimRFst  GainFGLUst=RGainFGLUst  GainFHAMst=RGainFHAMst  phiHATref=phiHATref  GainPhiHATHFLst=RGainPhiHATHFLst  GainDphiHATHFLst=RGainDphiHATHFLst  GainPhiHATGLUst=RGainPhiHATGLUst  GainDphiHATGLUst=RGainDphiHATGLUst  GainSGLUHAMst=RGainSGLUHAMst  GainSGLUcHFLst=RGainSGLUcHFLst  GainSHAMcHFLst=RGainSHAMcHFLst  GainSHFLcGLUst=RGainSHFLcGLUst  GainSRFcGLUst=RGainSRFcGLUst
  "R Stance, Swing, Trans (coronal)" : NeuroMuscularLibrary/Stance, Swing, Trans (coronal)  transSupst_C=RtransSupst_C  transsw_C=Rtranssw_C
  "R Stance, Swing, Trans amp (sagittal)" : NeuroMuscularLibrary/Stance, Swing, Trans amp (sagittal)  transSupst=RtransSupst  transsw=Rtranssw
  R Swing Phase (coronal) : NeuroMuscularLibrary/Swing Phase (coronal)  PreStimHABsw=RPreStimHABsw  PreStimHADsw=RPreStimHADsw  GainLHABsw=RGainLHABsw  GainLHADsw=RGainLHADsw
  R Swing Phase amp (sagittal) : NeuroMuscularLibrary/Swing Phase amp (sagittal)  PreStimHFLsw=RPreStimHFLsw  PreStimGLUsw=RPreStimGLUsw  PreStimHAMsw=RPreStimHAMsw  PreStimRFsw=RPreStimRFsw  GainLRFHFLsw=RGainLRFHFLsw  GainVRFHFLsw=RGainVRFHFLsw  GainLHAMGLUsw=RGainLHAMGLUsw  GainVHAMGLUsw=RGainVHAMGLUsw  GainLHAMsw=RGainLHAMsw  GainLHFLsw=RGainLHFLsw  GainLGLUsw=RGainLGLUsw  legLengthClr=RlegLengthClr  deltaLegAngleThr=RdeltaLegAngleThr
  Right Hard Stops : NeuroMuscularLibrary/Hard Stops  SystemSampleTime=-1  Latency=0  AutoFrameSizeCalculation=off
  SDelay{,3,6..9,12,14,16..19,29..30,32..33,36,38..39,41..42,47} (22 alike) : TransportDelay  DelayTime=ShortDelay
  SDelay{1..2,4..5,10..11,13,15,34,44..45,49} (12 alike) : TransportDelay  DelayTime=ShortDelay  InitialOutput=1
  SDelay20 : TransportDelay  DelayTime=ShortDelay  InitialOutput=LPreStimHFLinit
  SDelay21 : TransportDelay  DelayTime=ShortDelay  InitialOutput=LPreStimGLUinit
  SDelay22 : TransportDelay  DelayTime=ShortDelay  InitialOutput=LPreStimHAMinit
  SDelay23 : TransportDelay  DelayTime=ShortDelay  InitialOutput=LPreStimRFinit
  SDelay24 : TransportDelay  DelayTime=ShortDelay  InitialOutput=RPreStimHFLinit
  SDelay25 : TransportDelay  DelayTime=ShortDelay  InitialOutput=RPreStimGLUinit
  SDelay26 : TransportDelay  DelayTime=ShortDelay  InitialOutput=RPreStimHAMinit
  SDelay27 : TransportDelay  DelayTime=ShortDelay  InitialOutput=RPreStimRFinit
  SDelay35 : TransportDelay  DelayTime=ShortDelay  InitialOutput=RPreStimHABinit
  SDelay37 : TransportDelay  DelayTime=ShortDelay  InitialOutput=RPreStimHADinit
  SDelay40 : TransportDelay  DelayTime=ShortDelay  InitialOutput=LPreStimHADinit
  SDelay43 : TransportDelay  DelayTime=(ShortDelay + LongLoopDelay/2)  InitialOutput=LTargetAngleRInit
  SDelay46 : TransportDelay  DelayTime=ShortDelay  InitialOutput=LPreStimHABinit
  SDelay48 : TransportDelay  DelayTime=(ShortDelay + LongLoopDelay/2)  InitialOutput=RTargetAngleRInit
  Saturation{1..3,10} (4 alike) : Saturate  UpperLimit=1  LowerLimit=0.01  ZeroCross=off
  Selector : Selector  InputPortWidth=2  IndexOptions=Index vector (dialog)  Indices=[1]  OutputSizes=1
  Selector1 : Selector  InputPortWidth=2  IndexOptions=Index vector (dialog)  Indices=[1]  OutputSizes=1
  Selector2 : Selector  InputPortWidth=2  IndexOptions=Index vector (dialog)  Indices=[1]  OutputSizes=1
  Sum1 : Sum  Inputs=-+|
  Sum2 : Sum  Inputs=++|
  Sum3 : Sum  Inputs=--+
  Sum4 : Sum  Inputs=++|
  Sum5 : Sum  Inputs=--+
  Sum6 : Sum  Inputs=-+|
  TDelay28 : TransportDelay  DelayTime=(ShortDelay + LongLoopDelay/2)  InitialOutput=LTargetAngleInit
  TDelay31 : TransportDelay  DelayTime=(ShortDelay + LongLoopDelay/2)  InitialOutput=RTargetAngleInit
  hipM{1,4,9,12} (4 alike) : Selector  InputPortWidth=2  IndexOptions=Index vector (dialog)  Indices=1  OutputSizes=1
  hipM10 : Selector  InputPortWidth=3  IndexOptions=Index vector (dialog)  Indices=2  OutputSizes=1
  hipM{2,5,8,11} (4 alike) : Selector  InputPortWidth=3  IndexOptions=Index vector (dialog)  Indices=1  OutputSizes=1
  hipM3 : Selector  InputPortWidth=2  IndexOptions=Index vector (dialog)  Indices=2  OutputSizes=1
  hipM6 : Selector  InputPortWidth=2  IndexOptions=Index vector (dialog)  Indices=2  OutputSizes=1
  hipM7 : Selector  InputPortWidth=3  IndexOptions=Index vector (dialog)  Indices=2  OutputSizes=1
  tag scope: LAnkleMoment=global, LAnkleStopMoment=global, LHSwStim=global, LHipMoment=global, LHipMomentR=global, LHipRStopMoment=global, LHipStopMoment=global, LKneeMoment=global, LKneeStopMoment=global, LStimBFSH=global, LStimGAS=global, LStimGLU=global, LStimHAB=global, LStimHAD=global, LStimHAM=global, LStimHFL=global, LStimRF=global, LStimSOL=global, LStimTA=global, LStimVAS=global, RAnkleMoment=global, RAnkleStopMoment=global, RHSwStim=global, RHipMoment=global, RHipMomentR=global, RHipRStopMoment=global, RHipStopMoment=global, RKneeMoment=global, RKneeStopMoment=global, RStimBFSH=global, RStimGAS=global, RStimGLU=global, RStimHAB=global, RStimHAD=global, RStimHAM=global, RStimHFL=global, RStimRF=global, RStimSOL=global, RStimTA=global, RStimVAS=global, R_LHSwStim=global, R_RHSwStim=global
  wires:
  L Swing Phase (sagittal)/7 -> "L Stance, Swing, Trans (sagittal)"/18, hipM8/1
  Mux/1 -> [LHSwStim]
  hipM2/1 -> Add3/2
  SDelay11/1 -> L Swing Phase (sagittal)/11
  [RLceRF] -> SDelay4/1
  MDelay19/1 -> "L Stance, Swing, Trans (sagittal)"/2
  SDelay10/1 -> L Swing Phase (sagittal)/10
  hipM10/1 -> Add2/2
  R Stance Phase amp (sagittal)/5 -> "R Stance, Swing, Trans amp (sagittal)"/10
  hipM4/1 -> Add9/1
  SDelay2/1 -> L Swing Phase (sagittal)/5
  [RLceGLU] -> SDelay13/1
  L Swing Phase (sagittal)/1 -> "L Stance, Swing, Trans (sagittal)"/12
  LDelay/1 -> L Stance Phase (sagittal)/7
  L Stance Phase (sagittal)/1 -> "L Stance, Swing, Trans (sagittal)"/6
  SDelay9/1 -> L Swing Phase (sagittal)/6
  L Swing Phase (sagittal)/3 -> "L Stance, Swing, Trans (sagittal)"/14, hipM6/1, hipM4/1
  R Swing Phase amp (sagittal)/4 -> "R Stance, Swing, Trans amp (sagittal)"/14, hipM11/1
  Add2/1 -> Mux1/2
  L Swing Phase (sagittal)/5 -> "L Stance, Swing, Trans (sagittal)"/16
  SDelay14/1 -> "R Stance, Swing, Trans amp (sagittal)"/5
  R Stance Phase amp (sagittal)/2 -> "R Stance, Swing, Trans amp (sagittal)"/7
  SDelay12/1 -> "L Stance, Swing, Trans (sagittal)"/5
  MDelay2/1 -> L Stance Phase (sagittal)/5
  hipM6/1 -> Add1/1
  R Stance Phase amp (sagittal)/3 -> "R Stance, Swing, Trans amp (sagittal)"/8
  L Stance Phase (sagittal)/6 -> "L Stance, Swing, Trans (sagittal)"/11
  SDelay4/1 -> R Swing Phase amp (sagittal)/3
  hipM11/1 -> Mux1/4
  MDelay8/1 -> L Swing Phase (sagittal)/8
  Add3/1 -> Mux1/1
  R Swing Phase amp (sagittal)/3 -> "R Stance, Swing, Trans amp (sagittal)"/13, hipM12/1
  "R Stance, Swing, Trans amp (sagittal)"/1 -> Saturation1/1
  Add1/1 -> Mux/2
  hipM9/1 -> Mux/3
  L Stance Phase (sagittal)/3 -> "L Stance, Swing, Trans (sagittal)"/8
  Demux7/8 -> Multiply1/1
  Logical Operator2/1 -> R Swing Phase amp (sagittal)/Enable
  hipM5/1 -> Add9/2
  MDelay20/1 -> "L Stance, Swing, Trans (sagittal)"/1
  L Swing Phase (sagittal)/2 -> "L Stance, Swing, Trans (sagittal)"/13
  hipM8/1 -> Mux/4
  L Swing Phase (sagittal)/4 -> "L Stance, Swing, Trans (sagittal)"/15
  L Swing Phase (sagittal)/8 -> "L Stance, Swing, Trans (sagittal)"/19, hipM5/1, hipM7/1
  [LStance] -> MDelay20/1
  R Stance Phase amp (sagittal)/4 -> "R Stance, Swing, Trans amp (sagittal)"/9
  LL Delay3/1 -> SDelay30/1
  SDelay30/1 -> R Stance Phase amp (sagittal)/1
  SDelay29/1 -> L Stance Phase (sagittal)/1
  hipM1/1 -> Add3/1
  R Swing Phase amp (sagittal)/5 -> "R Stance, Swing, Trans amp (sagittal)"/15, hipM2/1, hipM10/1
  [LLceGLU] -> SDelay11/1
  [RLceHFL] -> SDelay5/1
  L Stance Phase (sagittal)/2 -> "L Stance, Swing, Trans (sagittal)"/7
  R Stance Phase amp (sagittal)/1 -> "R Stance, Swing, Trans amp (sagittal)"/6
  [LLceVAS] -> MDelay5/1
  [LHSwStim] -> R Stance Phase amp (sagittal)/2
  SDelay/1 -> "L Stance, Swing, Trans (sagittal)"/4
  Demux7/6 -> Multiply3/1
  Add9/1 -> Mux/1
  [LLceHFL] -> SDelay10/1
  [LLLoad] -> SDelay14/1
  Saturation1/1 -> Demux7/1
  SDelay5/1 -> R Swing Phase amp (sagittal)/7
  [LFmSOL] -> LDelay1/1
  hipM12/1 -> Mux1/3
  [LonR] -> "R Stance, Swing, Trans amp (sagittal)"/3
  [LLLoad] -> SDelay/1
  L Stance Phase (sagittal)/4 -> "L Stance, Swing, Trans (sagittal)"/9
  hipM3/1 -> Add2/1
  R Swing Phase amp (sagittal)/1 -> "R Stance, Swing, Trans amp (sagittal)"/11
  L Stance Phase (sagittal)/5 -> "L Stance, Swing, Trans (sagittal)"/10
  SDelay3/1 -> "R Stance, Swing, Trans amp (sagittal)"/4
  SDelay19/1 -> R Swing Phase amp (sagittal)/6
  [RVceHAM] -> SDelay19/1
  SDelay18/1 -> R Swing Phase amp (sagittal)/4
  SDelay15/1 -> R Swing Phase amp (sagittal)/5
  [RLceHAM] -> SDelay15/1
  Demux7/7 -> Multiply2/1
  [LLceBFSH] -> MDelay3/1
  [RLLoad] -> SDelay3/1
  SDelay17/1 -> R Stance Phase amp (sagittal)/4
  [RStance] -> MDelay19/1
  MDelay4/1 -> L Swing Phase (sagittal)/9
  L Swing Phase (sagittal)/6 -> "L Stance, Swing, Trans (sagittal)"/17, hipM9/1
  Demux7/9 -> Multiply/1
  [LVceBFSH] -> MDelay4/1
  SDelay8/1 -> L Swing Phase (sagittal)/4
  [RVceRF] -> SDelay18/1
  MDelay5/1 -> L Swing Phase (sagittal)/12
  SDelay16/1 -> R Stance Phase amp (sagittal)/3
  [RLLoad] -> SDelay12/1
  R Swing Phase amp (sagittal)/2 -> "R Stance, Swing, Trans amp (sagittal)"/12, hipM3/1, hipM1/1
  [LVceRF] -> SDelay8/1
  SDelay13/1 -> R Swing Phase amp (sagittal)/8
  Mux1/1 -> [RHSwStim]
  L Stance afferent delay/1 -> L Stance Phase (sagittal)/Enable, Logical Operator/1
  Logical Operator3/1 -> L Swing Phase (sagittal)/Enable
  [LLceRF] -> SDelay1/1
  [LVceHAM] -> SDelay9/1
  LDelay2/1 -> L Stance Phase (sagittal)/9
  [LLceTA] -> LDelay2/1
  SDelay1/1 -> L Swing Phase (sagittal)/3
  [RFmHAM] -> SDelay17/1
  Logical Operator/1 -> Logical Operator3/2
  [LLceHAM] -> SDelay2/1
  LDelay1/1 -> L Stance Phase (sagittal)/8
  [LFmGAS] -> LDelay/1
  [RFmGLU] -> SDelay16/1
  MDelay3/1 -> L Stance Phase (sagittal)/6
  SDelay6/1 -> L Stance Phase (sagittal)/3
  [LVceVAS] -> MDelay8/1
  [LFmVAS] -> MDelay2/1
  LL Delay2/1 -> SDelay29/1
  [LFmGLU] -> SDelay6/1
  SDelay7/1 -> L Stance Phase (sagittal)/4
  Demux7/5 -> Multiply4/1
  [LFmHAM] -> SDelay7/1
  [RHSwStim] -> L Stance Phase (sagittal)/2
  hipM7/1 -> Add1/2
  Logical Operator1/1 -> Logical Operator2/2
  [LLceTA] -> LDelay13/1
  MDelay17/1 -> L Swing Phase (sagittal)/7
  [LLceBFSH] -> MDelay17/1
  LDelay13/1 -> L Swing Phase (sagittal)/13
  R Stance afferent delay/1 -> R Swing Phase amp (sagittal)/1, R Stance Phase amp (sagittal)/Enable, Logical Operator1/1
  [RonL] -> "L Stance, Swing, Trans (sagittal)"/3
  [LonR] -> Logical Operator2/1
  [RonL] -> Logical Operator3/1
  [RStance] -> MDelay13/1
  MDelay13/1 -> "R Stance, Swing, Trans amp (sagittal)"/1
  [LStance] -> MDelay14/1
  MDelay14/1 -> "R Stance, Swing, Trans amp (sagittal)"/2
  [Ralpha_tgt] -> Sum1/2
  Selector/1 -> Sum6/1, Sum1/1
  [Lalpha_tgt] -> Sum6/2
  [phiANDdphiHAT] -> LL Delay2/1, LL Delay3/1
  [RFmHAB] -> SDelay38/1
  SDelay35/1 -> [RStimHAB]
  [LFmHAB] -> SDelay39/1
  SDelay37/1 -> [RStimHAD]
  [LLceHAD] -> SDelay44/1
  SDelay39/1 -> L Stance Phase (coronal)/4
  L Stance Phase (coronal)/2 -> "L Stance, Swing, Trans (coronal)"/7
  MDelay21/1 -> "L Stance, Swing, Trans (coronal)"/2
  L Swing Phase (coronal)/2 -> "L Stance, Swing, Trans (coronal)"/11, Sum2/2
  [LhipR_tgt] -> Sum3/2
  L GLU Golgi Tendon Organs2/1 -> Sum3/1
  Logical Operator5/1 -> Logical Operator6/2
  [RLceHAD] -> SDelay49/1
  Selector2/1 -> L GLU Golgi Tendon Organs2/1
  Logical Operator4/1 -> Logical Operator7/2
  [LLceHAB] -> SDelay45/1
  Constant4/1 -> R Stance Phase (coronal)/1
  [RonL] -> Logical Operator7/1
  Logical Operator6/1 -> R Swing Phase (coronal)/Enable
  L Swing Phase (coronal)/1 -> "L Stance, Swing, Trans (coronal)"/10, Sum2/1
  L Stance Phase (coronal)/1 -> "L Stance, Swing, Trans (coronal)"/6
  SDelay32/1 -> "L Stance, Swing, Trans (coronal)"/4
  L GLU Golgi Tendon Organs1/1 -> LL Delay6/1
  "L Stance, Swing, Trans (coronal)"/1 -> Saturation3/1
  SDelay43/1 -> L Swing Phase (coronal)/1
  MDelay24/1 -> "L Stance, Swing, Trans (coronal)"/1
  Selector1/1 -> Sum5/1
  L Stance afferent delay1/1 -> Logical Operator4/1, L Stance Phase (coronal)/Enable
  SDelay46/1 -> [LStimHAB]
  Sum3/1 -> SDelay43/1
  SDelay45/1 -> L Swing Phase (coronal)/3
  SDelay44/1 -> L Swing Phase (coronal)/2
  [RStance] -> MDelay23/1
  MDelay23/1 -> "R Stance, Swing, Trans (coronal)"/1
  SDelay49/1 -> R Swing Phase (coronal)/2
  [R_LHSwStim] -> R Stance Phase (coronal)/3
  Sum5/1 -> SDelay48/1
  Logical Operator7/1 -> L Swing Phase (coronal)/Enable
  Sum2/1 -> [R_LHSwStim]
  [LStance] -> L Stance afferent delay1/1
  L Stance Phase (coronal)/4 -> "L Stance, Swing, Trans (coronal)"/9
  SDelay42/1 -> L Stance Phase (coronal)/2
  [RonL] -> "L Stance, Swing, Trans (coronal)"/3
  L Stance afferent delay2/1 -> R Stance Phase (coronal)/Enable, Logical Operator5/1
  L Stance Phase (coronal)/3 -> "L Stance, Swing, Trans (coronal)"/8
  SDelay36/1 -> "L Stance, Swing, Trans (coronal)"/5
  [LLLoad] -> SDelay32/1
  [RStance] -> MDelay21/1
  [RLLoad] -> SDelay33/1
  [RStance] -> L Stance afferent delay2/1
  [LStance] -> MDelay24/1
  [LLLoad] -> SDelay41/1
  [LonR] -> Logical Operator6/1
  [RLLoad] -> SDelay36/1
  [R_RHSwStim] -> L Stance Phase (coronal)/3
  L GLU Golgi Tendon Organs3/1 -> L Stance Phase (coronal)/1
  SDelay41/1 -> "R Stance, Swing, Trans (coronal)"/5
  "R Stance, Swing, Trans (coronal)"/1 -> Saturation2/1
  SDelay47/1 -> R Stance Phase (coronal)/2
  R Stance Phase (coronal)/2 -> "R Stance, Swing, Trans (coronal)"/7
  SDelay38/1 -> R Stance Phase (coronal)/4
  Saturation2/1 -> Demux1/1
  [LStance] -> MDelay22/1
  SDelay34/1 -> R Swing Phase (coronal)/3
  MDelay22/1 -> "R Stance, Swing, Trans (coronal)"/2
  [LonR] -> "R Stance, Swing, Trans (coronal)"/3
  SDelay48/1 -> R Swing Phase (coronal)/1
  [RLceHAB] -> SDelay34/1
  R Stance Phase (coronal)/1 -> "R Stance, Swing, Trans (coronal)"/6
  Saturation3/1 -> Demux2/1
  R Swing Phase (coronal)/1 -> "R Stance, Swing, Trans (coronal)"/10, Sum4/1
  LL Delay7/1 -> SDelay47/1
  R Stance Phase (coronal)/3 -> "R Stance, Swing, Trans (coronal)"/8
  LL Delay6/1 -> SDelay42/1
  R Stance Phase (coronal)/4 -> "R Stance, Swing, Trans (coronal)"/9
  R Swing Phase (coronal)/2 -> "R Stance, Swing, Trans (coronal)"/11, Sum4/2
  SDelay33/1 -> "R Stance, Swing, Trans (coronal)"/4
  Sum4/1 -> [R_RHSwStim]
  [RhipR_tgt] -> Sum5/2
  Constant3/1 -> L GLU Golgi Tendon Organs3/1
  "L Stance, Swing, Trans (sagittal)"/1 -> Saturation10/1
  [RphiANDdphiHip] -> Right Hard Stops/2
  Demux10/2 -> Multiply8/1
  [RphiANDdphiAnkle] -> Right Hard Stops/4
  [LMuscleTorques] -> Left Hard Stops/1
  [LphiANDdphiAnkle] -> Left Hard Stops/4
  [LphiANDdphiKnee] -> Left Hard Stops/3
  [RMuscleTorques] -> Right Hard Stops/1
  [LphiANDdphiHip] -> Left Hard Stops/2
  Right Hard Stops/1 -> Demux10/1
  Left Hard Stops/1 -> Demux8/1
  Right Hard Stops/3 -> Multiply6/1
  Demux10/1 -> [RHipMoment]
  Demux10/3 -> Multiply7/1
  Left Hard Stops/4 -> [LAnkleStopMoment]
  Right Hard Stops/2 -> [RHipStopMoment]
  Left Hard Stops/3 -> [LKneeStopMoment]
  Right Hard Stops/4 -> Multiply5/1
  Demux8/2 -> [LKneeMoment]
  Left Hard Stops/2 -> [LHipStopMoment]
  Demux8/1 -> [LHipMoment]
  Demux8/3 -> [LAnkleMoment]
  [RphiANDdphiKnee] -> Right Hard Stops/3
  [LMuscleTorquesR] -> Left Hard Stops/5
  [RMuscleTorquesR] -> Right Hard Stops/5
  Left Hard Stops/5 -> [LHipMomentR]
  Right Hard Stops/5 -> [RHipMomentR]
  [LthetaANDdthetaHipR] -> Left Hard Stops/6
  [RthetaANDdthetaHipR] -> Right Hard Stops/6
  Left Hard Stops/6 -> [LHipRStopMoment]
  Right Hard Stops/6 -> [RHipRStopMoment]
  [phiANDdphiHAT] -> Selector/1
  [thetaANDdthetaHAT] -> LL Delay7/1, Selector1/1
  [thetaANDdthetaHAT] -> L GLU Golgi Tendon Organs1/1, Selector2/1
  [LStance] -> L Swing Phase (sagittal)/1, L Stance afferent delay/1
  [RStance] -> R Stance afferent delay/1
  Multiply/1 -> [RStimTA]
  Multiply1/1 -> [RStimSOL]
  Multiply2/1 -> [RStimGAS]
  Multiply3/1 -> [RStimBFSH]
  Multiply4/1 -> [RStimVAS]
  [RlegLength] -> R Swing Phase amp (sagittal)/9
  Multiply5/1 -> [RAnkleStopMoment]
  Multiply6/1 -> [RKneeStopMoment]
  Multiply7/1 -> [RAnkleMoment]
  Multiply8/1 -> [RKneeMoment]
  Saturation10/1 -> Demux6/1
  LDelay10/1 -> [LStimTA]
  LDelay9/1 -> [LStimSOL]
  Demux6/3 -> SDelay22/1
  Demux6/9 -> LDelay10/1
  Demux6/8 -> LDelay9/1
  Demux6/7 -> LDelay11/1
  Demux6/5 -> MDelay9/1
  Demux6/2 -> SDelay21/1
  SDelay20/1 -> [LStimHFL]
  SDelay22/1 -> [LStimHAM]
  Demux6/4 -> SDelay23/1
  MDelay9/1 -> [LStimVAS]
  LDelay11/1 -> [LStimGAS]
  MDelay10/1 -> [LStimBFSH]
  Demux6/1 -> SDelay20/1
  SDelay23/1 -> [LStimRF]
  Demux6/6 -> MDelay10/1
  SDelay21/1 -> [LStimGLU]
  Demux7/2 -> SDelay25/1
  SDelay24/1 -> [RStimHFL]
  Demux7/3 -> SDelay26/1
  SDelay26/1 -> [RStimHAM]
  Demux7/1 -> SDelay24/1
  SDelay27/1 -> [RStimRF]
  Demux7/4 -> SDelay27/1
  SDelay25/1 -> [RStimGLU]
  TDelay31/1 -> R Swing Phase amp (sagittal)/2
  Sum1/1 -> TDelay31/1
  Sum6/1 -> TDelay28/1
  TDelay28/1 -> L Swing Phase (sagittal)/2
  Demux2/1 -> SDelay46/1
  Demux2/2 -> SDelay40/1
  SDelay40/1 -> [LStimHAD]
  Demux1/2 -> SDelay37/1
  Demux1/1 -> SDelay35/1
  Constant1/1 -> Sum5/3
  Constant2/1 -> Sum3/3
